simulink model "curentul_rotoric"  (R2022b)
settings: Solver=VariableStepAuto  StartTime=0.0  StopTime=10.0  RelTol=1e-3
values from neighbouring files (symbols this model uses):
  k = 0.035    [date_indrumator.m]    (also in proiect.m)
settings Model: Creator=Ruxandra  LastModifiedBy=Ruxandra

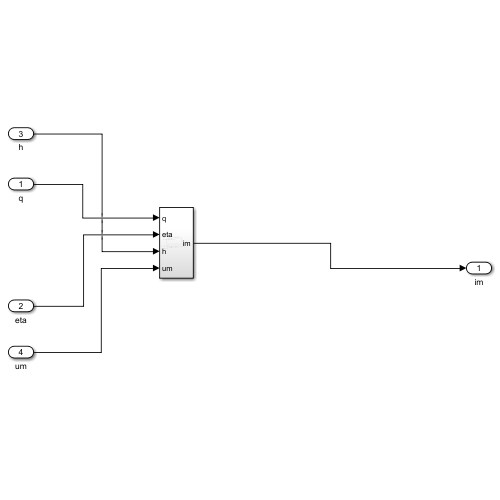
[thumbnail: Simulink's stored preview of the top-level diagram]
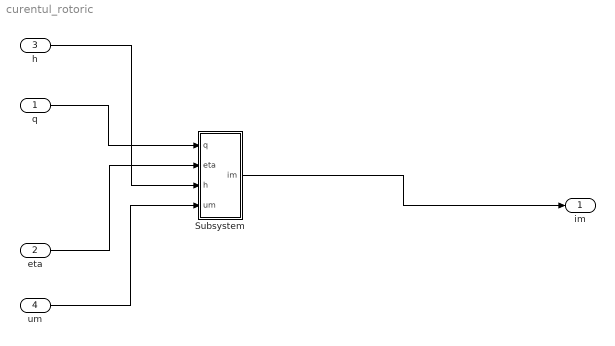
== system curentul_rotoric ==
  q : Inport
  eta : Inport  Port=2
  h : Inport  Port=3
  um : Inport  Port=4
  Subsystem : Subsystem
  im : Outport
  wires:
  q/1 -> Subsystem/1(q)
  eta/1 -> Subsystem/2(eta)
  h/1 -> Subsystem/3(h)
  um/1 -> Subsystem/4(um)
  Subsystem/1(im) -> im/1

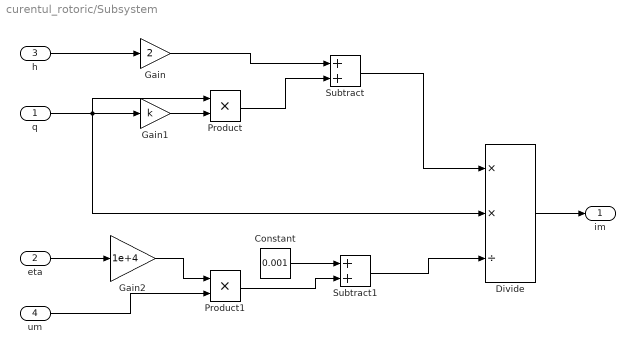
== system curentul_rotoric/Subsystem ==
  q : Inport
  eta : Inport  Port=2
  h : Inport  Port=3
  um : Inport  Port=4
  Constant : Constant  Value=0.001
  Divide : Product  Inputs=**/
  Gain : Gain  Gain=2
  Gain1 : Gain  Gain=k
  Gain2 : Gain  Gain=1e+4
  Product : Product
  Product1 : Product
  Subtract : Sum
  Subtract1 : Sum
  im : Outport
  wires:
  Product/1 -> Subtract/2
  h/1 -> Gain/1
  Gain/1 -> Subtract/1
  Subtract1/1 -> Divide/3
  Gain2/1 -> Product1/1
  Constant/1 -> Subtract1/1
  Subtract/1 -> Divide/1
  Gain1/1 -> Product/2
  eta/1 -> Gain2/1
  Product1/1 -> Subtract1/2
  q/1 -> Divide/2, Gain1/1, Product/1
  um/1 -> Product1/2
  Divide/1 -> im/1
